simulink model "keg_mealy2"  (R2015a)
settings: Solver=ode45  StartTime=0.0  StopTime=500  RelTol=1e-3
undefined symbols (not defined in the file): sigbuilder_block
settings Model: Creator=lenovo  LastModifiedBy=lenovo

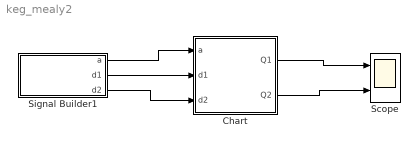
== system keg_mealy2 ==
  Chart : Stateflow chart  TreatAsAtomicUnit=on
  Scope : Scope  NumInputPorts=2
      settings: YMin=-5~-5  YMax=5~5
  Signal Builder1 : Subsystem  Tag=STV Subsys  LoadFcn=sigbuilder_block('load');  StartFcn=sigbuilder_block('start');  StopFcn=sigbuilder_block('stop');  ClipboardFcn=sigbuilder_block('clipboard');  mask(Sigbuilder block){}
      mask help: Simulink:masks:SigbuilderBlock_MD
      mask init:
      | if ~strcmp(get_param(bdroot(gcbh),'SimulationStatus'),'stopped') tuvar = sigbuilder_block('maskInit'); end
      settings: CopyFcn=sigbuilder_block('copy');  DeleteFcn=sigbuilder_block('delete');  ModelCloseFcn=sigbuilder_block('modelClose');  PreSaveFcn=sigbuilder_block('preSave');  PauseFcn=sigbuilder_block('pause');  ContinueFcn=sigbuilder_block('continue');  NameChangeFcn=sigbuilder_block('namechange');  OpenFcn=sigbuilder_block('open',[198.75 94.5 550.5 399.75 ]);  CloseFcn=sigbuilder_block('close');
      mask Display: plot(0, 0, 100, 100,[2, 2, 32, 32, 2], [68, 8, 8, 68, 68],[32, 2], [38, 38], [32, 19, 2],[53, 60, 44], [32, 17, 17, 2],[16, 16, 31, 31]);txt = getActiveGroup(gcbh);text(2, 100, txt,'verticalAlignment', 'top');
  wires:
  Chart/1(Q1) -> Scope/1
  Chart/2(Q2) -> Scope/2
  Signal Builder1/1(a) -> Chart/1(a)
  Signal Builder1/2(d1) -> Chart/2(d1)
  Signal Builder1/3(d2) -> Chart/3(d2)

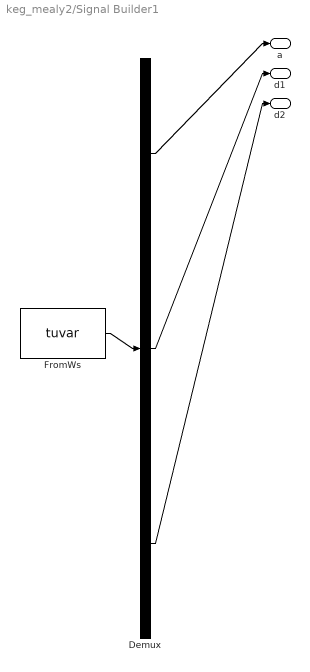
== system keg_mealy2/Signal Builder1 ==
  Demux : Demux  Tag=STV Demux  Outputs=3
  FromWs : FromWorkspace  Tag=STV FromWs  VariableName=tuvar  SampleTime=0
      SigBuilderData=|
      | common.afterFinalStr = 'Extrapolate'
      | common.sampleTime = 0
      | dataSet.timeRange = [0 500]
      | dataSet.name = 'Group 1'
      | sbobj.Groups.Name = 'Group 1'
      | sbobj.Groups.Signals(1).Name = 'a'
      | sbobj.Groups.Signals(1).XData = [0 7 7 42 42 47 47 100 100 106 106 150 150 155 155 206 206 214 214 257 257 266 266 300 300 304 304 350 350 354 354 400 400 403 403 450 450 454 454 500]
      | sbobj.Groups.Signals(1).YData = [1 1 0 0 1 1 0 0 1 1 0 0 1 1 0 0 1 1 0 0 1 1 0 0 1 1 0 0 1 1 0 0 1 1 0 0 1 1 0 0]
      | sbobj.Groups.Signals(2).Name = 'd1'
      | sbobj.Groups.Signals(2).XData = [0 25 62 62 68 68 100 111 178 178 186 186 200 225 250 250 257 257 300 333 333 339 339 415 415 424 424 450 475 475 481 481 500]
      | sbobj.Groups.Signals(2).YData = [0 0 0 1 1 0 0 0 0 1 1 0 0 0 0 1 1 0 0 0 1 1 0 0 1 1 0 0 0 1 1 0 0]
      | sbobj.Groups.Signals(3).Name = 'd2'
      | sbobj.Groups.Signals(3).XData = [0 25 50 75 100 100 106 106 150 175 200 200 205 205 250 275 293 293 299 299 350 375 392 392 399 399 450 475 487 487 494 494 500]
      | sbobj.Groups.Signals(3).YData = [0 0 0 0 0 1 1 0 0 0 0 1 1 0 0 0 0 1 1 0 0 0 0 1 1 0 0 0 0 1 1 0 0]
      | sbobj.Groups.TimeRange = [0 500]
  a : Outport  Tag=STV Outport
  d1 : Outport  Tag=STV Outport  Port=2
  d2 : Outport  Tag=STV Outport  Port=3
  wires:
  Demux/1 -> a/1
  Demux/2 -> d1/1
  Demux/3 -> d2/1
  FromWs/1 -> Demux/1

== stateflow chart keg_mealy2/Chart ==
  settings: stateMachineType=MEALY_MACHINE
  state 01
  state 00
  state 21
  state 10
  state 11
  10 -> 11 [order 3] : [a==1&d1==1]{Q1=1;Q2=1}
  11 -> 10 [order 1] : [d2==1&d1==0]{Q1=1;Q2=0}
  11 -> 11 [order 4] : [d1==1&d2==1&a==1]{Q1=1;Q2=1}
  (default) -> 00
  10 -> 01 [order 1] : [d1==1&a==0]{Q1=0;Q2=1}
  11 -> 21 [order 3] : [d1==1&d2==0]{Q1=2;Q2=1}
  00 -> 10 : [a==1]{Q1=1;Q2=0}
  01 -> 11 [order 2] : [a==1]{Q1=1;Q2=1}
  01 -> 10 [order 3] : [a==1&d2==1]{Q1=1;Q2=0}
  21 -> 11 [order 2] : [a==1&d2==1]{Q1=1;Q2=1}
  11 -> 01 [order 5] : [d2==1&a==0]{Q1=0;Q2=1}
  10 -> 10 [order 2] : [a==1]{Q1=1;Q2=0}
  01 -> 00 [order 1] : [a==0&d2==1]{Q1=0;Q2=0}
  21 -> 01 [order 1] : [d2==1&a==0]{Q1=0;Q2=1}
  11 -> 11 [order 2] : [a==1]{Q1=1;Q2=1}
  data: a input; d1 input; d2 input; Q1 output; Q2 output
